simulink model "GFM_GFL_referenceModel_abcCoordinates"  (R2023b)
settings: Solver=ode23  StartTime=0.0  StopTime=SimulationSetup.Solver.timeSimulationEnd  MaxStep=SimulationSetup.Solver.MaxStep  RelTol=SimulationSetup.Solver.RelTol
undefined symbols (not defined in the file): freq, H, Ibase, K_damping, Kdroop_V, Ki_CC, ki_P, ki_PLL, ki_Q, Kp_CC, kp_P, kp_PLL, kp_Q, Lconv1, Lg, Lv, Qref, Rconv1, Rg, Rv, Sbase, SimulationSetup, Vpeak, wf_PQ, wg
libraries: spsPower3phInstantaneousLib x4, eeTransforms x2, eeStairGenerator x1
settings Model: Creator=kauchr  LastModifiedBy=kauchr
settings DataIOCC: SaveFinalState=on  SaveOperatingPoint=on  SaveState=on

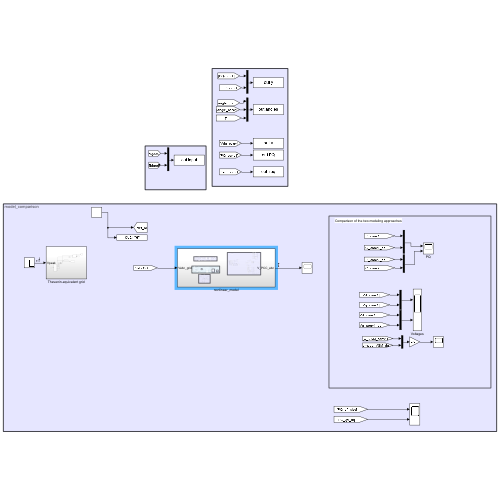
[thumbnail: Simulink's stored preview of the top-level diagram]
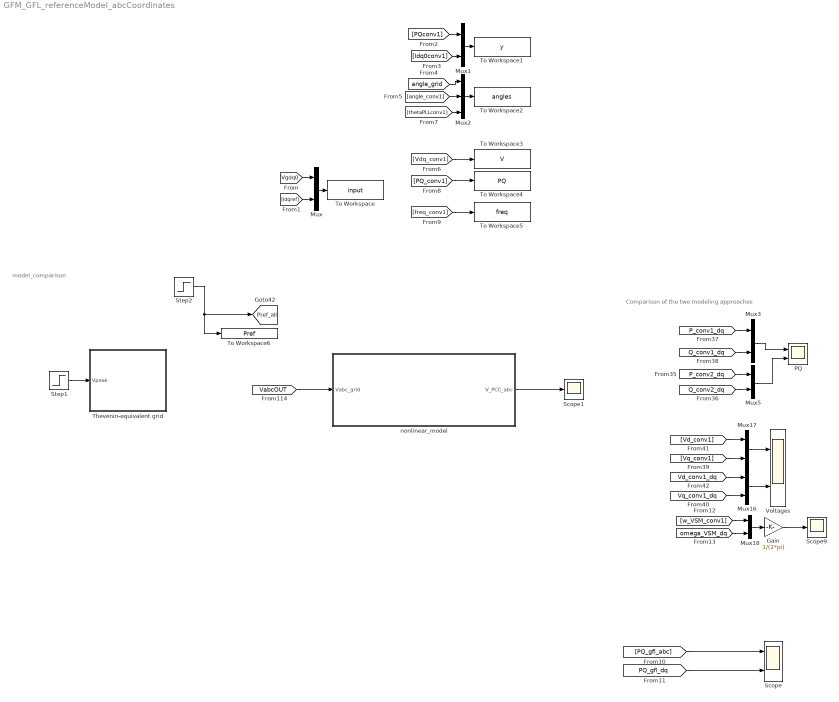
== system GFM_GFL_referenceModel_abcCoordinates ==
  note: model_comparison
  note: Comparison of the two modeling approaches
  Gain : Gain  Gain=1/(2*pi)
  Mux{,1,3,5,16..18} (7 alike) : Mux  Inputs=2
  Mux2 : Mux  Inputs=3
  PQ : Scope  NumInputPorts=2
  Scope : Scope  NumInputPorts=2
  Scope1 : Scope
  Scope9 : Scope
  Step1 : Step  Time=SimulationSetup.grid.voltageAmplitudeStep.Time  Before=SimulationSetup.grid.voltageAmplitudeStep.Values(1)  After=SimulationSetup.grid.voltageAmplitudeStep.Values(2)  SampleTime=0
  Step2 : Step  Time=SimulationSetup.converter1.Pref.Time  Before=SimulationSetup.converter1.Pref.Values(1)  After=SimulationSetup.converter1.Pref.Values(2)  SampleTime=0
  Thevenin-equivalent grid : Subsystem
  To Workspace : ToWorkspace  VariableName=input  SaveFormat=Timeseries  SampleTime=-1
  To Workspace1 : ToWorkspace  VariableName=y  SaveFormat=Timeseries  SampleTime=-1
  To Workspace2 : ToWorkspace  VariableName=angles  SaveFormat=Timeseries  SampleTime=-1
  To Workspace3 : ToWorkspace  VariableName=V  SaveFormat=Timeseries  SampleTime=-1
  To Workspace4 : ToWorkspace  VariableName=PQ  SaveFormat=Timeseries  SampleTime=-1
  To Workspace5 : ToWorkspace  VariableName=freq  SaveFormat=Timeseries  SampleTime=-1
  To Workspace6 : ToWorkspace  VariableName=Pref  SaveFormat=Timeseries  SampleTime=-1
      settings: Save2DSignal=2-D array (concatenate along first dimension)
  Voltages : Scope  NumInputPorts=2
  nonlinear_model : Subsystem
  tag scope: Pref_all=global
  wires:
  [Vgdq0] -> Mux/1
  [Idqref] -> Mux/2
  Mux/1 -> To Workspace/1
  Mux1/1 -> To Workspace1/1
  [PQconv1] -> Mux1/1
  [Idq0conv1] -> Mux1/2
  Mux2/1 -> To Workspace2/1
  [angle_grid] -> Mux2/1
  [angle_conv1] -> Mux2/2
  [Vdq_conv1] -> To Workspace3/1
  [thetaPLLconv1] -> Mux2/3
  [PQ_conv1] -> To Workspace4/1
  [freq_conv1] -> To Workspace5/1
  nonlinear_model/1(V_PCC_abc) -> Scope1/1
  [VabcOUT] -> nonlinear_model/1(Vabc_grid)
  [PQ_gfl_dq] -> Scope/2
  [PQ_gfl_abc] -> Scope/1
  [Vq_conv1] -> Mux17/2
  [Vd_conv1_dq] -> Mux16/1
  [Vq_conv1_dq] -> Mux16/2
  [Vd_conv1] -> Mux17/1
  [P_conv1_dq] -> Mux3/1
  [Q_conv1_dq] -> Mux3/2
  Mux5/1 -> PQ/2
  [Q_conv2_dq] -> Mux5/2
  [P_conv2_dq] -> Mux5/1
  Mux3/1 -> PQ/1
  Gain/1 -> Scope9/1
  Mux18/1 -> Gain/1
  [omega_VSM_dq] -> Mux18/2
  [w_VSM_conv1] -> Mux18/1
  Mux17/1 -> Voltages/1
  Mux16/1 -> Voltages/2
  Step1/1 -> Thevenin-equivalent grid/1(Vpeak)
  Step2/1 -> [Pref_all], To Workspace6/1

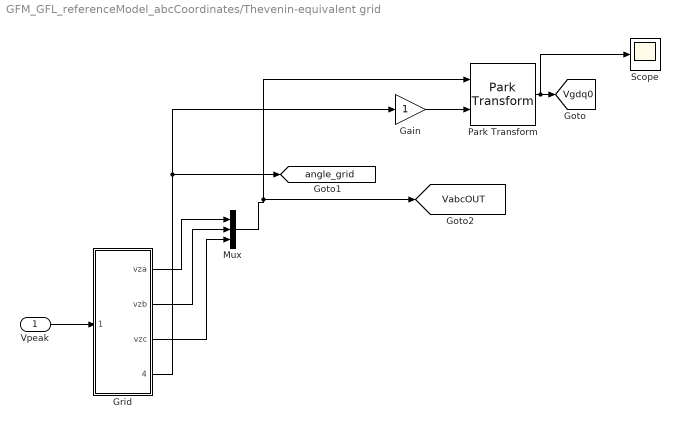
== system GFM_GFL_referenceModel_abcCoordinates/Thevenin-equivalent grid ==
  Vpeak : Inport
  Gain : Gain
  Grid : Subsystem
  Mux : Mux  Inputs=3
  Park Transform : eeTransforms/Park Transform  AxisAlignment=D-axis  PowerInvariant=off
      settings: LibrarySourceBlock=|
      | ee_sl_lib/Mathematical
      | Transforms/Park Transform
  Scope : Scope
  tag scope: VabcOUT=global, Vgdq0=global, angle_grid=global
  wires:
  Grid/4(thetareal) -> [angle_grid], Gain/1
  Grid/2(vzb) -> Mux/2
  Grid/3(vzc) -> Mux/3
  Mux/1 -> Park Transform/1, [VabcOUT]
  Park Transform/1 -> Scope/1, [Vgdq0]
  Grid/1(vza) -> Mux/1
  Vpeak/1 -> Grid/1(Vpeak)
  Gain/1 -> Park Transform/2

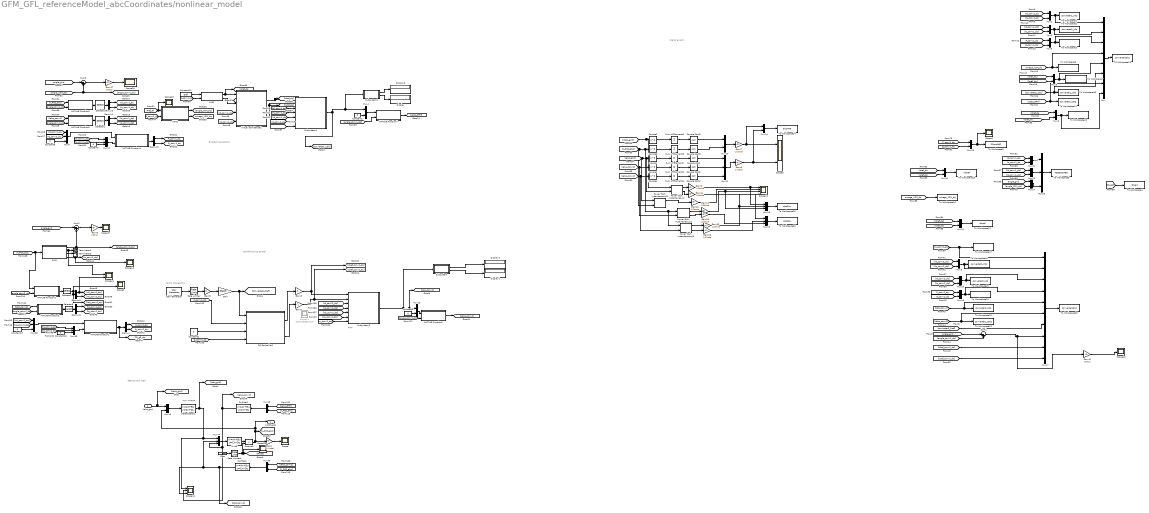
== system GFM_GFL_referenceModel_abcCoordinates/nonlinear_model ==
  note: Grid-forming Control
  note: sign!
  note: had to change this
  note: sign omega
  note: Grid-following Control
  note: Signal export
  note: Network and load
  Vabc_grid : Inport
  AVR2 : Subsystem
  Constant{1..3,6..7,16..17} (7 alike) : Constant  Value=0
  Constant11 : Constant  Value=Qref
  Demux{,1..3,5..6} (6 alike) : Demux  Outputs=2
  Display{,1..3} (4 alike) : Display
  Gain : Gain  Gain=Sbase
  Gain{9..10,12..16} (7 alike) : Gain  Gain=1/Sbase
  Gain11 : Gain  Gain=180/pi
  Gain17 : Gain  Gain=180/pi
  Gain2 : Gain  Gain=-1
  Gain3 : Gain
  Gain4 : Gain  Gain=1/Vpeak
  Gain5 : Gain
  Gain6 : Gain  Gain=180/pi
  Gain7 : Gain  Gain=1/Vpeak
  Gain8 : Gain  Gain=1/Ibase
  MATLAB Function1 : MATLAB Function  TreatAsAtomicUnit=on
  MATLAB Function2 : MATLAB Function  TreatAsAtomicUnit=on
  MATLAB Function3 : MATLAB Function  TreatAsAtomicUnit=on
  MATLAB Function4 : MATLAB Function  TreatAsAtomicUnit=on
  MATLAB Function5 : MATLAB Function  TreatAsAtomicUnit=on
  MATLAB Function6 : MATLAB Function  TreatAsAtomicUnit=on
  MATLAB Function7 : MATLAB Function  TreatAsAtomicUnit=on
  MATLAB Function8 : MATLAB Function  TreatAsAtomicUnit=on
  Mux : Mux  Inputs=[2 2 2 1 2 2 3 2]
  Mux{1..3,5..6,9..10,15..16,21,23..24,29..31} (15 alike) : Mux  Inputs=2
  Mux{8,11..12,18..19,25,38..39} (8 alike) : Mux  Inputs=3
  Mux13 : Mux  Inputs=[2 1]
  Mux14 : Mux  Inputs=[2 3]
  Mux17 : Mux  Inputs=[1 2 2 2 2 3 1 1 1 1]
  Mux4 : Mux  Inputs=[2 1]
  Mux43 : Mux  Inputs=[3 3]
  Mux44 : Mux  Inputs=[3 3 3]
  Mux45 : Mux  Inputs=[3 3]
  Mux46 : Mux  Inputs=[3 3]
  PLL3 : Subsystem
  PQ-Controller2 : Subsystem
  Power (3ph, Instantaneous){,1..3} (4 alike) : spsPower3phInstantaneousLib/Power (3ph, Instantaneous)
  Product1 : Product
  RL-filter1 : StateSpace  A=-Rconv1/Lconv1*eye(3)  B=1/Lconv1*[eye(3),- eye(3)]  C=eye(3)  D=zeros(3,6)  InitialCondition=0
  RL-filter2 : StateSpace  A=-Rconv1/Lconv1*eye(3)  B=1/Lconv1*[eye(3),- eye(3)]  C=eye(3)  D=zeros(3,6)  InitialCondition=0
  Rate Limiter : RateLimiter  RisingSlewLimit=100  FallingSlewLimit=-100  SampleTimeMode=inherited
  Rate Limiter1 : RateLimiter  RisingSlewLimit=1000000  FallingSlewLimit=-1000000  SampleTimeMode=inherited
  Rvirt3 : StateSpace  A=[]  B=[]  C=[]  D=[eye(3),eye(3),eye(3)]  InitialCondition=0  ContinuousStateAttributes='VDQ_PCC'
  Scope{,1,10,13,15..18} (8 alike) : Scope
  Scope11 : Scope  NumInputPorts=3
  Scope12 : Scope  NumInputPorts=4
  Scope14 : Scope  Commented=on  NumInputPorts=2
  Scope2 : Scope  NumInputPorts=2
  Scope24 : Scope  NumInputPorts=2
  Scope3 : Scope  NumInputPorts=2
  Selector{,1..3} (4 alike) : Selector  InputPortWidth=3  IndexOptions=Index vector (dialog)  Indices=[1 2]  OutputSizes=1
  Square{,1..4} (5 alike) : Math  Operator=square
  Square Root{,1..4} (5 alike) : Sqrt
  Stair Generator : eeStairGenerator/Stair Generator  LabelModeActiveChoice=Continuous  TimeInput=SimulationSetup.converter2.Pref.Time  AmplitudeInput=SimulationSetup.converter2.Pref.Values  SampleTime=0  RepeatPattern=off  OutDataTypeStr=double
      settings: LibrarySourceBlock=ee_sl_lib/General Control/Stair Generator
  State-Space1 : StateSpace  A=-Rg/Lg*eye(3)  B=1/Lg*[eye(3),- eye(3)]  C=eye(3)  D=zeros(3,6)  InitialCondition=0
  Step : Step  Time=SimulationSetup.Load.Step.Time  Before=SimulationSetup.Load.Base  After=SimulationSetup.Load.Step.Value  SampleTime=0
  Subsystem : Subsystem
  Subsystem1 : Subsystem
  Subsystem2 : Subsystem
  Subsystem3 : Subsystem
  Sum of Elements{,1..4} (5 alike) : Sum  Inputs=+
  Sum1 : Sum  Inputs=|-+
  Sum2 : Sum  Inputs=|-+
  Sum3 : Sum  Inputs=|-+
  Terminator4 : Terminator
  Terminator5 : Terminator
  To Workspace1 : ToWorkspace  VariableName=converter1_Vdq  SaveFormat=Structure With Time  SampleTime=-1
  To Workspace10 : ToWorkspace  VariableName=Vdqref  SaveFormat=Timeseries  SampleTime=-1
      settings: Save2DSignal=2-D array (concatenate along first dimension)
  To Workspace11 : ToWorkspace  VariableName=Idqref  SaveFormat=Timeseries  SampleTime=-1
      settings: Save2DSignal=2-D array (concatenate along first dimension)
  To Workspace12 : ToWorkspace  VariableName=omega_VSM_dq  SaveFormat=Timeseries  SampleTime=-1
      settings: Save2DSignal=2-D array (concatenate along first dimension)
  To Workspace13 : ToWorkspace  VariableName=converter1_Udq  SaveFormat=Timeseries  SampleTime=-1
      settings: Save2DSignal=2-D array (concatenate along first dimension)
  To Workspace14 : ToWorkspace  VariableName=converter1_UDQ  SaveFormat=Timeseries  SampleTime=-1
      settings: Save2DSignal=2-D array (concatenate along first dimension)
  To Workspace15 : ToWorkspace  VariableName=converter1_Vdrefqref  SaveFormat=Timeseries  SampleTime=-1
      settings: Save2DSignal=2-D array (concatenate along first dimension)
  To Workspace16 : ToWorkspace  VariableName=converter1abc  SaveFormat=Structure With Time  SampleTime=-1
  To Workspace17 : ToWorkspace  VariableName=converter2_omegaPLL  SaveFormat=Timeseries  SampleTime=-1
      settings: Save2DSignal=2-D array (concatenate along first dimension)
  To Workspace18 : ToWorkspace  VariableName=converter2_Vdq  SaveFormat=Structure With Time  SampleTime=-1
  To Workspace19 : ToWorkspace  VariableName=converter2_Idq  SaveFormat=Structure With Time  SampleTime=-1
  To Workspace2 : ToWorkspace  VariableName=converter1_Idq  SaveFormat=Structure With Time  SampleTime=-1
  To Workspace20 : ToWorkspace  VariableName=converter2_PmeasQmeas  SaveFormat=Structure With Time  SampleTime=-1
  To Workspace21 : ToWorkspace  VariableName=converter2_Udq  SaveFormat=Timeseries  SampleTime=-1
      settings: Save2DSignal=2-D array (concatenate along first dimension)
  To Workspace22 : ToWorkspace  VariableName=converter2_Uabc  SaveFormat=Timeseries  SampleTime=-1
      settings: Save2DSignal=2-D array (concatenate along first dimension)
  To Workspace23 : ToWorkspace  VariableName=converter2abc  SaveFormat=Structure  SampleTime=-1
      settings: Save2DSignal=2-D array (concatenate along first dimension)
  To Workspace24 : ToWorkspace  VariableName=abcMAG  SaveFormat=Structure  SampleTime=-1
      settings: Save2DSignal=2-D array (concatenate along first dimension)
  To Workspace25 : ToWorkspace  VariableName=abcPpu  SaveFormat=Structure  SampleTime=-1
      settings: Save2DSignal=2-D array (concatenate along first dimension)
  To Workspace26 : ToWorkspace  VariableName=abcQpu  SaveFormat=Structure  SampleTime=-1
      settings: Save2DSignal=2-D array (concatenate along first dimension)
  To Workspace3 : ToWorkspace  VariableName=converter1_PmeasQmeas  SaveFormat=Structure With Time  SampleTime=-1
  To Workspace4 : ToWorkspace  VariableName=Rload  SaveFormat=Timeseries  SampleTime=-1
      settings: Save2DSignal=2-D array (concatenate along first dimension)
  To Workspace5 : ToWorkspace  VariableName=testDataABC  SaveFormat=Structure With Time  SampleTime=-1
  To Workspace6 : ToWorkspace  VariableName=converter1_omegaVSM  SaveFormat=Timeseries  SampleTime=-1
      settings: Save2DSignal=2-D array (concatenate along first dimension)
  To Workspace7 : ToWorkspace  VariableName=converter1_IdrefIqref  SaveFormat=Timeseries  SampleTime=-1
      settings: Save2DSignal=2-D array (concatenate along first dimension)
  To Workspace9 : ToWorkspace  VariableName=PQoutABC  SaveFormat=Timeseries  SampleTime=-1
      settings: Save2DSignal=2-D array (concatenate along first dimension)
  VSM2 : Subsystem
  Virtual admittance1 : Subsystem
  V_PCC_abc : Outport
  tag scope: PQ_gfl_dq=global, P_conv1_dq=global, P_conv2_dq=global, Q_conv1_dq=global, Q_conv2_dq=global, Vd_conv1_dq=global, Vdref_dq=global, Vq_conv1_dq=global, Vqref_dq=global, omega_VSM_dq=global
  wires:
  [Id_conv1_dq] -> Subsystem1/3(Id)
  Mux24/1 -> Mux25/3
  [Pref_all] -> Scope18/1, VSM2/1(Pref)
  Mux29/1 -> Scope1/1, To Workspace9/1
  Mux30/1 -> To Workspace10/1
  Demux3/2 -> [Q_conv1_dq]
  Constant6/1 -> Mux8/3
  AVR2/1(Vdref) -> [Vdref_dq], Virtual admittance1/1(Vdref)
  [P_conv1_dq] -> VSM2/2(Pmeas)
  [Iq_conv1_dq] -> Mux23/2
  Demux3/1 -> [P_conv1_dq]
  [Vq_conv1_dq] -> Subsystem1/6(Vq)
  [angle_VSM_dq] -> Mux24/2
  Mux31/1 -> To Workspace11/1
  Sum3/1 -> Gain17/1
  [Q_conv1_dq] -> Mux29/2
  [Vd_conv1_dq] -> Mux8/1
  Mux8/1 -> MATLAB Function4/1(Vdq0)
  Constant7/1 -> Mux12/3
  Constant11/1 -> AVR2/1(Qref)
  Virtual admittance1/1(Idref) -> [Idref_dq], Subsystem1/1(Idref)
  [Vq_conv1_dq] -> Mux21/2
  AVR2/2(Vqref) -> [Vqref_dq], Virtual admittance1/2(Vqref)
  Demux1/1 -> [Id_conv1_dq]
  [Id_conv1_dq] -> Mux12/1
  [omega_VSM_dq] -> Subsystem1/7(omega)
  VSM2/1(angle_VSM) -> [angle_VSM_dq]
  [Vq_conv1_dq] -> Mux8/2
  Demux2/2 -> [Vq_conv1_dq]
  Demux1/2 -> [Iq_conv1_dq]
  [Iqref_dq] -> Mux31/2
  [Vd_conv1_dq] -> Subsystem1/5(Vd)
  [Vdref_dq] -> Mux30/1
  [omega_VSM_dq] -> To Workspace12/1
  [Vd_conv1_dq] -> Virtual admittance1/3(Vd)
  [angle_grid] -> Sum3/1
  Demux2/1 -> [Vd_conv1_dq]
  [Q_conv1_dq] -> AVR2/2(Qmeas)
  [Vq_conv1_dq] -> Virtual admittance1/4(Vq)
  Mux23/1 -> Mux25/2
  [Iq_conv1_dq] -> Subsystem1/4(Iq)
  [angle_grid] -> Mux24/1
  [Id_conv1_dq] -> Mux23/1
  Mux21/1 -> Mux25/1
  [Vd_conv1_dq] -> Mux21/1
  [Iq_conv1_dq] -> Mux12/2
  VSM2/2(omega_VSM) -> [omega_VSM_dq]
  [Idref_dq] -> Mux31/1
  Mux25/1 -> To Workspace5/1
  [Vqref_dq] -> Mux30/2
  Virtual admittance1/2(Iqref) -> Subsystem1/2(Iqref), [Iqref_dq]
  [P_conv1_dq] -> Mux29/1
  Subsystem1/1(Uconv_dq) -> [converter1_Udq], Subsystem2/1(dq), Mux4/1
  [Vd_conv2_dq] -> Mux38/1
  MATLAB Function1/1(y) -> [PQ_gfl_dq], Demux/1
  Constant17/1 -> Mux38/3
  Mux38/1 -> MATLAB Function1/1(Vdq0)
  PLL3/2(Vd) -> Scope24/1, Terminator4/1
  Demux6/1 -> [Id_conv2_dq]
  Demux5/2 -> [Vq_conv2_dq]
  [P_conv2_dq] -> PQ-Controller2/2(Pmeas)
  Constant16/1 -> Mux39/3
  Selector2/1 -> [Vdq_conv2_dq], Demux5/1, Scope2/2
  PLL3/1(angle) -> Sum2/2, [angle_conv2_dq]
  [Id_conv2_dq] -> Subsystem3/3(Id)
  [Vq_conv2_dq] -> Mux38/2
  [Id_conv2_dq] -> Mux39/1
  [Iq_conv2_dq] -> Mux39/2
  [Iq_conv2_dq] -> Subsystem3/4(Iq)
  [Q_conv2_dq] -> PQ-Controller2/4(Qmeas)
  PLL3/3(Vq) -> Terminator5/1
  [Vd_conv2_dq] -> Subsystem3/5(Vd)
  [Vq_conv2_dq] -> Subsystem3/6(Vq)
  Demux5/1 -> Scope24/2, [Vd_conv2_dq]
  PLL3/4(w_grid) -> Scope13/1, [w_conv2_dq]
  Demux6/2 -> [Iq_conv2_dq]
  Mux39/1 -> MATLAB Function1/2(Idq0)
  Mux45/1 -> State-Space1/1
  Mux43/1 -> RL-filter2/1
  RL-filter2/1 -> Mux44/3, Scope11/2, [Iabc_conv1]
  [V_PCC_abc] -> Mux46/2
  [Uabc_conv2] -> Mux46/1
  State-Space1/1 -> [Iabc_grid], Scope11/1, Mux44/1
  Mux46/1 -> RL-filter1/1
  Mux44/1 -> Rvirt3/1
  [Uabc_GFM] -> Mux43/1
  [V_PCC_abc] -> Mux43/2
  [w_conv2_dq] -> Subsystem3/7(omega)
  Mux1/1 -> Mux/1, To Workspace1/1
  [Vq_conv1_dq] -> Mux1/2
  [Vd_conv1_dq] -> Mux1/1
  [Iq_conv1_dq] -> Mux2/2
  [Id_conv1_dq] -> Mux2/1
  Mux3/1 -> Mux/3, To Workspace3/1
  [Q_conv1_dq] -> Mux3/2
  [P_conv1_dq] -> Mux3/1
  [omega_VSM_dq] -> Mux/4, To Workspace6/1
  [Idref_dq] -> Mux5/1
  [Iqref_dq] -> Mux5/2
  Mux5/1 -> Mux/5, To Workspace7/1
  [converter1_Udq] -> Mux/6, To Workspace13/1
  [Uabc_GFM] -> Mux/7, To Workspace14/1
  Mux6/1 -> To Workspace15/1, Mux/8
  [Vqref_dq] -> Mux6/2
  [Vdref_dq] -> Mux6/1
  Mux2/1 -> Mux/2, To Workspace2/1
  Mux/1 -> To Workspace16/1
  [w_conv2_dq] -> Mux17/1, To Workspace17/1
  [Vd_conv2_dq] -> Mux9/1
  Mux9/1 -> Mux17/2, To Workspace18/1
  Mux15/1 -> Mux17/3, To Workspace19/1
  [P_conv2_dq] -> Mux16/1
  [Vq_conv2_dq] -> Mux9/2
  Mux16/1 -> Mux17/4, To Workspace20/1
  [Q_conv2_dq] -> Mux16/2
  [Iq_conv2_dq] -> Mux15/2
  [Id_conv2_dq] -> Mux15/1
  [Udq_conv2] -> Mux17/5, To Workspace21/1
  [Uabc_conv2] -> Mux17/6, To Workspace22/1
  Mux17/1 -> To Workspace23/1
  Vabc_grid/1 -> [Vabc_grid], Mux45/1
  Selector3/1 -> Demux6/1
  [V_PCC_abc] -> MATLAB Function5/1(Vabc)
  [angle_conv1_dq] -> MATLAB Function5/2(theta)
  Selector1/1 -> Demux1/1
  [Iabc_conv1] -> MATLAB Function6/1(Vabc)
  [angle_conv1_dq] -> MATLAB Function6/2(theta)
  Selector/1 -> Demux2/1
  Stair Generator/1 -> Rate Limiter/1
  PQ-Controller2/1(Idref) -> Gain3/1
  PQ-Controller2/2(Iqref) -> Gain2/1
  Gain3/1 -> [Idref_conv2_dq], Subsystem3/1(Idref)
  Gain2/1 -> Subsystem3/2(Iqref), [Iqref_conv2_dq]
  Constant2/1 -> PQ-Controller2/3(Qref)
  [converter2_Pref] -> Mux17/7
  Rate Limiter/1 -> Gain5/1
  RL-filter1/1 -> Mux44/2, Scope11/3, [Iabc_conv2]
  [Idref_conv2_dq] -> Mux17/9
  [Iqref_conv2_dq] -> Mux17/10
  Rvirt3/1 -> Product1/1
  Product1/1 -> Gain4/1, Mux45/2, V_PCC_abc/1, [V_PCC_abc]
  Step/1 -> Rate Limiter1/1
  Gain4/1 -> Scope/1
  [Rload] -> To Workspace4/1
  Rate Limiter1/1 -> Product1/2, [Rload], Scope15/1
  Gain5/1 -> Gain/1
  Gain6/1 -> Scope17/1
  Gain7/1 -> Mux14/1, Scope3/1
  Square Root3/1 -> Mux10/2  "load"
  Square Root1/1 -> Mux11/2  "GFL"
  Square Root2/1 -> Mux10/1  "grid"
  Gain8/1 -> Mux14/2, Scope3/2
  [V_PCC_abc] -> "Power (3ph, Instantaneous)3"/1, "Power (3ph, Instantaneous)2"/1, Square3/1, "Power (3ph, Instantaneous)1"/2
  [Iabc_grid] -> "Power (3ph, Instantaneous)"/2, Square/1, "Power (3ph, Instantaneous)1"/1
  Sum of Elements3/1 -> Square Root3/1
  Square3/1 -> Sum of Elements3/1
  Square2/1 -> Sum of Elements2/1
  [Iabc_conv2] -> "Power (3ph, Instantaneous)2"/2, Square1/1
  Sum of Elements2/1 -> Square Root2/1
  Square Root/1 -> Mux11/1  "grid"
  Square1/1 -> Sum of Elements1/1
  Square/1 -> Sum of Elements/1
  Sum of Elements/1 -> Square Root/1
  Mux11/1 -> Gain8/1
  [Vabc_grid] -> "Power (3ph, Instantaneous)"/1, Square2/1
  Mux10/1 -> Gain7/1
  Sum of Elements1/1 -> Square Root1/1
  Square4/1 -> Sum of Elements4/1
  Sum of Elements4/1 -> Square Root4/1
  [Iabc_conv1] -> "Power (3ph, Instantaneous)3"/2, Square4/1
  Square Root4/1 -> Mux11/3  "GFM"
  MATLAB Function5/1(y) -> Selector/1
  MATLAB Function6/1(y) -> Selector1/1
  [angle_conv1_dq] -> MATLAB Function7/2(theta)
  Mux4/1 -> MATLAB Function7/1(Vdq0)
  Constant1/1 -> Mux4/2
  [angle_VSM_dq] -> [angle_conv1_dq], Sum3/2
  [angle_conv2_dq] -> MATLAB Function3/2(theta)
  [Iabc_conv2] -> MATLAB Function3/1(Iabc)
  MATLAB Function2/1(y) -> Selector2/1
  [angle_conv2_dq] -> MATLAB Function2/2(theta)
  MATLAB Function3/1(y) -> Selector3/1
  [V_PCC_abc] -> MATLAB Function2/1(Vabc), PLL3/1(Vabc)
  Constant3/1 -> Mux13/2
  [angle_conv2_dq] -> MATLAB Function8/2(theta)
  MATLAB Function8/1(Vabc) -> [Uabc_conv2]
  Mux13/1 -> MATLAB Function8/1(Vdq0)
  Mux14/1 -> To Workspace24/1
  [angle_grid] -> Sum1/1
  [angle_conv2_dq] -> Sum1/2
  Sum1/1 -> Gain11/1, Mux17/8
  "Power (3ph, Instantaneous)"/1 -> Gain9/1
  "Power (3ph, Instantaneous)1"/1 -> Gain10/1
  Gain9/1 -> Mux18/1, Scope12/1
  Gain10/1 -> Scope12/2
  Gain11/1 -> Scope10/1
  "Power (3ph, Instantaneous)2"/1 -> Gain12/1
  Gain12/1 -> Mux18/3, Scope12/3
  "Power (3ph, Instantaneous)3"/1 -> Gain13/1
  Gain13/1 -> Mux18/2, Scope12/4
  Mux18/1 -> To Workspace25/1
  "Power (3ph, Instantaneous)"/2 -> Gain14/1
  Mux19/1 -> To Workspace26/1
  Gain14/1 -> Mux19/1
  "Power (3ph, Instantaneous)2"/2 -> Gain15/1
  "Power (3ph, Instantaneous)3"/2 -> Gain16/1
  Gain16/1 -> Mux19/2
  Gain15/1 -> Mux19/3
  Subsystem3/1(Uconv_dq) -> Subsystem/1(dq), Mux13/1, [Udq_conv2]
  Subsystem/1(Vmag (pu)) -> Display2/1
  Subsystem/2(Angle (°)) -> Display1/1
  Subsystem2/2(Angle (°)) -> Display/1
  Subsystem2/1(Vmag (pu)) -> Display3/1
  Gain17/1 -> Scope16/1
  [angle_grid] -> Sum2/1
  Sum2/1 -> Gain6/1
  Gain/1 -> [converter2_Pref], PQ-Controller2/1(Pref)
  Demux/1 -> [P_conv2_dq]
  Demux/2 -> [Q_conv2_dq]
  Mux12/1 -> MATLAB Function4/2(Idq0)
  MATLAB Function4/1(y) -> Demux3/1
  MATLAB Function7/1(Vabc) -> [Uabc_GFM]

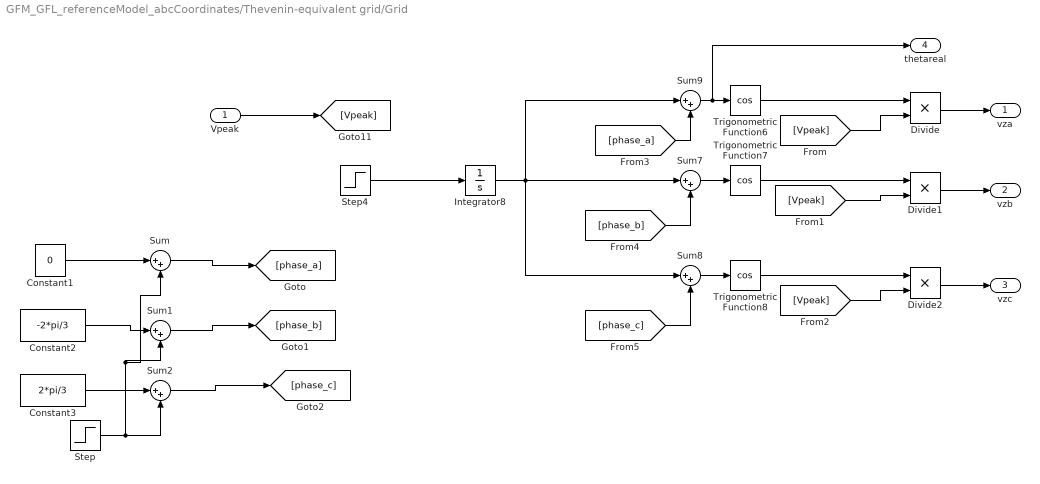
== system GFM_GFL_referenceModel_abcCoordinates/Thevenin-equivalent grid/Grid ==
  Vpeak : Inport
  Constant1 : Constant  Value=0
  Constant2 : Constant  Value=-2*pi/3
  Constant3 : Constant  Value=2*pi/3
  Divide : Product  Inputs=**
  Divide1 : Product  Inputs=**
  Divide2 : Product  Inputs=**
  Integrator8 : Integrator  ContinuousStateAttributes='grid_thetaGRID'
  Step : Step  Time=SimulationSetup.grid.PhaseStep.Time  Before=SimulationSetup.grid.PhaseStep.Values(1)  After=SimulationSetup.grid.PhaseStep.Values(2)  SampleTime=0
  Step4 : Step  Time=SimulationSetup.grid.FrequencyStep.Time  Before=SimulationSetup.grid.FrequencyStep.Values(1)  After=SimulationSetup.grid.FrequencyStep.Values(2)  SampleTime=0
  Sum{,1..2,7..9} (6 alike) : Sum  Inputs=|++
  Trigonometric Function6 : Trigonometry  Operator=cos
  Trigonometric Function7 : Trigonometry  Operator=cos
  Trigonometric Function8 : Trigonometry  Operator=cos
  vza : Outport
  vzb : Outport  Port=2
  vzc : Outport  Port=3
  thetareal : Outport  Port=4
  wires:
  Sum9/1 -> thetareal/1, Trigonometric Function6/1
  [phase_c] -> Sum8/2
  Integrator8/1 -> Sum8/1, Sum9/1, Sum7/1
  [phase_b] -> Sum7/2
  Sum7/1 -> Trigonometric Function7/1
  [phase_a] -> Sum9/2
  Sum8/1 -> Trigonometric Function8/1
  Trigonometric Function6/1 -> Divide/1
  Trigonometric Function7/1 -> Divide1/1
  Trigonometric Function8/1 -> Divide2/1
  Divide/1 -> vza/1
  Divide1/1 -> vzb/1
  Divide2/1 -> vzc/1
  [Vpeak] -> Divide/2
  [Vpeak] -> Divide1/2
  [Vpeak] -> Divide2/2
  Sum1/1 -> [phase_b]
  Sum/1 -> [phase_a]
  Constant1/1 -> Sum/1
  Constant2/1 -> Sum1/1
  Constant3/1 -> Sum2/1
  Sum2/1 -> [phase_c]
  Step/1 -> Sum/2, Sum1/2, Sum2/2
  Step4/1 -> Integrator8/1
  Vpeak/1 -> [Vpeak]

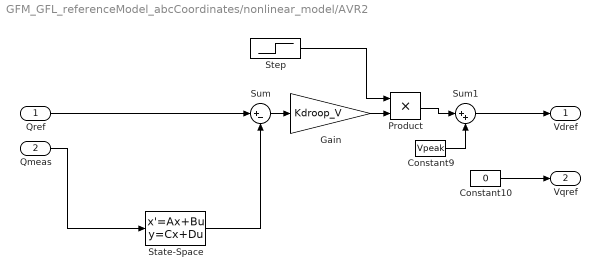
== system GFM_GFL_referenceModel_abcCoordinates/nonlinear_model/AVR2 ==
  Qref : Inport
  Qmeas : Inport  Port=2
  Constant10 : Constant  Value=0
  Constant9 : Constant  Value=Vpeak
  Gain : Gain  Gain=Kdroop_V
  Product : Product
  State-Space : StateSpace  A=-wf_PQ  B=wf_PQ  D=0  InitialCondition=0  ContinuousStateAttributes='converter1_xI_Vdroop'
  Step : Step  Time=SimulationSetup.converter1.VoltageCtrl.ActivationTime  SampleTime=0
  Sum : Sum  Inputs=|+-
  Sum1 : Sum  Inputs=|++
  Vdref : Outport
  Vqref : Outport  Port=2
  wires:
  Qref/1 -> Sum/1
  Constant9/1 -> Sum1/2
  Sum/1 -> Gain/1
  Qmeas/1 -> State-Space/1
  Product/1 -> Sum1/1
  Step/1 -> Product/1
  Gain/1 -> Product/2
  State-Space/1 -> Sum/2
  Sum1/1 -> Vdref/1
  Constant10/1 -> Vqref/1

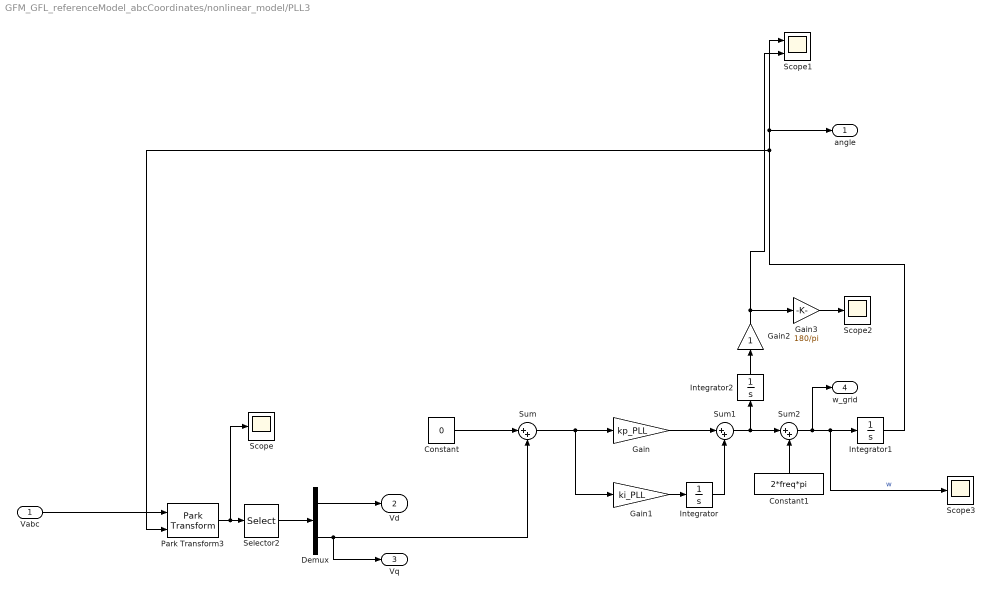
== system GFM_GFL_referenceModel_abcCoordinates/nonlinear_model/PLL3 ==
  Vabc : Inport
  Constant : Constant  Value=0
  Constant1 : Constant  Value=2*freq*pi
  Demux : Demux  Outputs=2
  Gain : Gain  Gain=kp_PLL
  Gain1 : Gain  Gain=ki_PLL
  Gain2 : Gain
  Gain3 : Gain  Gain=180/pi
  Integrator : Integrator  ContinuousStateAttributes='converter2_xI_PLL'
  Integrator1 : Integrator  ContinuousStateAttributes='converter2_thetaPLL'
  Integrator2 : Integrator  ContinuousStateAttributes='converter2_deltaPLL'
  Park Transform3 : eeTransforms/Park Transform  AxisAlignment=D-axis  PowerInvariant=off
      settings: LibrarySourceBlock=|
      | ee_sl_lib/Mathematical
      | Transforms/Park Transform
  Scope : Scope
  Scope1 : Scope  NumInputPorts=2
  Scope2 : Scope
  Scope3 : Scope
  Selector2 : Selector  InputPortWidth=3  IndexOptions=Index vector (dialog)  Indices=[1 2]  OutputSizes=1
  Sum : Sum  Inputs=|++
  Sum1 : Sum  Inputs=|++
  Sum2 : Sum  Inputs=|++
  angle : Outport
  Vd : Outport  Port=2
  Vq : Outport  Port=3
  w_grid : Outport  Port=4
  wires:
  Sum1/1 -> Sum2/1, Integrator2/1
  Gain/1 -> Sum1/1
  Integrator/1 -> Sum1/2
  Gain1/1 -> Integrator/1
  Demux/1 -> Vd/1
  Sum2/1 -> w_grid/1, Scope3/1, Integrator1/1  "w"
  Constant/1 -> Sum/1
  Constant1/1 -> Sum2/2
  Vabc/1 -> Park Transform3/1
  Sum/1 -> Gain1/1, Gain/1
  Demux/2 -> Sum/2, Vq/1
  Integrator2/1 -> Gain2/1
  Integrator1/1 -> Park Transform3/2, angle/1, Scope1/1
  Gain2/1 -> Gain3/1, Scope1/2
  Park Transform3/1 -> Scope/1, Selector2/1
  Selector2/1 -> Demux/1
  Gain3/1 -> Scope2/1

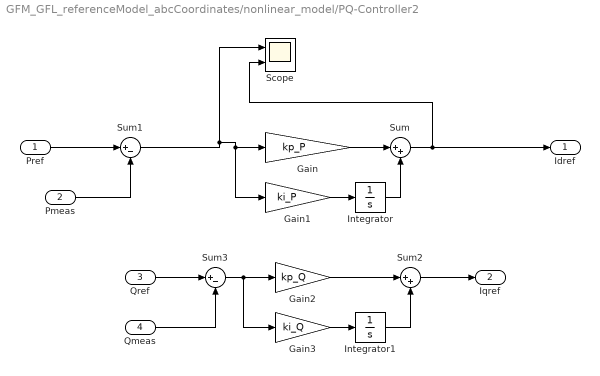
== system GFM_GFL_referenceModel_abcCoordinates/nonlinear_model/PQ-Controller2 ==
  Pref : Inport
  Pmeas : Inport  Port=2
  Qref : Inport  Port=3
  Qmeas : Inport  Port=4
  Gain : Gain  Gain=kp_P
  Gain1 : Gain  Gain=ki_P
  Gain2 : Gain  Gain=kp_Q
  Gain3 : Gain  Gain=ki_Q
  Integrator : Integrator  ContinuousStateAttributes='converter2_xI_Pctrl'
  Integrator1 : Integrator  ContinuousStateAttributes='converter2_xI_Qctrl'
  Scope : Scope  NumInputPorts=2
  Sum : Sum  Inputs=|++
  Sum1 : Sum  Inputs=|+-
  Sum2 : Sum  Inputs=|++
  Sum3 : Sum  Inputs=|+-
  Idref : Outport
  Iqref : Outport  Port=2
  wires:
  Gain1/1 -> Integrator/1
  Integrator/1 -> Sum/2
  Gain/1 -> Sum/1
  Sum/1 -> Idref/1, Scope/2
  Pmeas/1 -> Sum1/2
  Integrator1/1 -> Sum2/2
  Sum2/1 -> Iqref/1
  Sum3/1 -> Gain3/1, Gain2/1
  Gain2/1 -> Sum2/1
  Qmeas/1 -> Sum3/2
  Gain3/1 -> Integrator1/1
  Qref/1 -> Sum3/1
  Sum1/1 -> Scope/1, Gain1/1, Gain/1
  Pref/1 -> Sum1/1

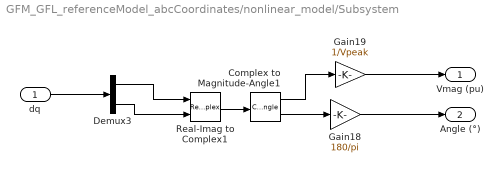
== system GFM_GFL_referenceModel_abcCoordinates/nonlinear_model/Subsystem ==
  dq : Inport
  Complex to Magnitude-Angle1 : ComplexToMagnitudeAngle
  Demux3 : Demux  Outputs=2
  Gain18 : Gain  Gain=180/pi
  Gain19 : Gain  Gain=1/Vpeak
  Real-Imag to Complex1 : RealImagToComplex
  Vmag (pu) : Outport
  Angle (°) : Outport  Port=2
  wires:
  Demux3/2 -> Real-Imag to Complex1/2
  Complex to Magnitude-Angle1/1 -> Gain19/1
  dq/1 -> Demux3/1
  Gain19/1 -> Vmag (pu)/1
  Complex to Magnitude-Angle1/2 -> Gain18/1
  Real-Imag to Complex1/1 -> Complex to Magnitude-Angle1/1
  Gain18/1 -> Angle (°)/1
  Demux3/1 -> Real-Imag to Complex1/1

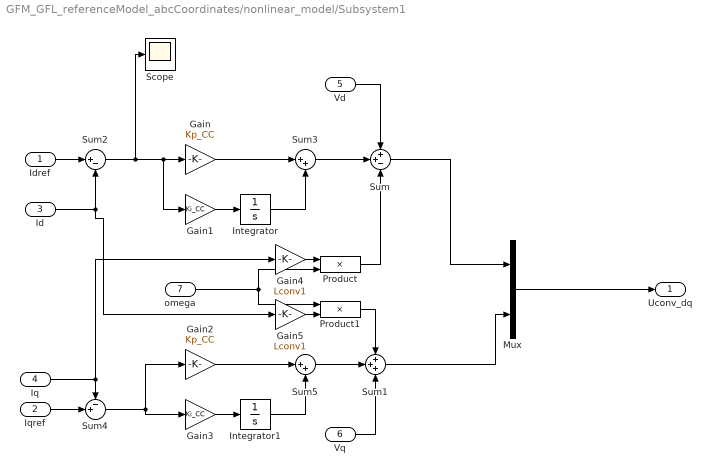
== system GFM_GFL_referenceModel_abcCoordinates/nonlinear_model/Subsystem1 ==
  Idref : Inport
  Iqref : Inport  Port=2
  Id : Inport  Port=3
  Iq : Inport  Port=4
  Vd : Inport  Port=5
  Vq : Inport  Port=6
  omega : Inport  Port=7
  Gain : Gain  Gain=Kp_CC
  Gain1 : Gain  Gain=Ki_CC
  Gain2 : Gain  Gain=Kp_CC
  Gain3 : Gain  Gain=Ki_CC
  Gain4 : Gain  Gain=Lconv1
  Gain5 : Gain  Gain=Lconv1
  Integrator : Integrator  ContinuousStateAttributes='converter1_xId_CC'
  Integrator1 : Integrator  ContinuousStateAttributes='converter1_xIq_CC'
  Mux : Mux  Inputs=2
  Product : Product
  Product1 : Product
  Scope : Scope
  Sum : Sum  Inputs=++-
  Sum1 : Sum  Inputs=+++
  Sum2 : Sum  Inputs=|+-
  Sum3 : Sum  Inputs=|++
  Sum4 : Sum  Inputs=-+|
  Sum5 : Sum  Inputs=|++
  Uconv_dq : Outport
  wires:
  Vd/1 -> Sum/1
  Vq/1 -> Sum1/3
  Sum/1 -> Mux/1
  Sum1/1 -> Mux/2
  Mux/1 -> Uconv_dq/1
  Idref/1 -> Sum2/1
  Id/1 -> Sum2/2, Gain5/1
  Sum2/1 -> Scope/1, Gain1/1, Gain/1
  Gain1/1 -> Integrator/1
  Integrator/1 -> Sum3/2
  Gain/1 -> Sum3/1
  Sum3/1 -> Sum/2
  Iqref/1 -> Sum4/2
  Iq/1 -> Gain4/1, Sum4/1
  Integrator1/1 -> Sum5/2
  Sum5/1 -> Sum1/2
  Gain3/1 -> Integrator1/1
  Gain2/1 -> Sum5/1
  Sum4/1 -> Gain2/1, Gain3/1
  Gain4/1 -> Product/1
  Product/1 -> Sum/3
  omega/1 -> Product/2, Product1/1
  Gain5/1 -> Product1/2
  Product1/1 -> Sum1/1

== system GFM_GFL_referenceModel_abcCoordinates/nonlinear_model/Subsystem2 ==
  dq : Inport
  Complex to Magnitude-Angle1 : ComplexToMagnitudeAngle
  Demux3 : Demux  Outputs=2
  Gain18 : Gain  Gain=180/pi
  Gain19 : Gain  Gain=1/Vpeak
  Real-Imag to Complex1 : RealImagToComplex
  Vmag (pu) : Outport
  Angle (°) : Outport  Port=2
  wires:
  Demux3/2 -> Real-Imag to Complex1/2
  Complex to Magnitude-Angle1/1 -> Gain19/1
  dq/1 -> Demux3/1
  Gain19/1 -> Vmag (pu)/1
  Complex to Magnitude-Angle1/2 -> Gain18/1
  Real-Imag to Complex1/1 -> Complex to Magnitude-Angle1/1
  Gain18/1 -> Angle (°)/1
  Demux3/1 -> Real-Imag to Complex1/1

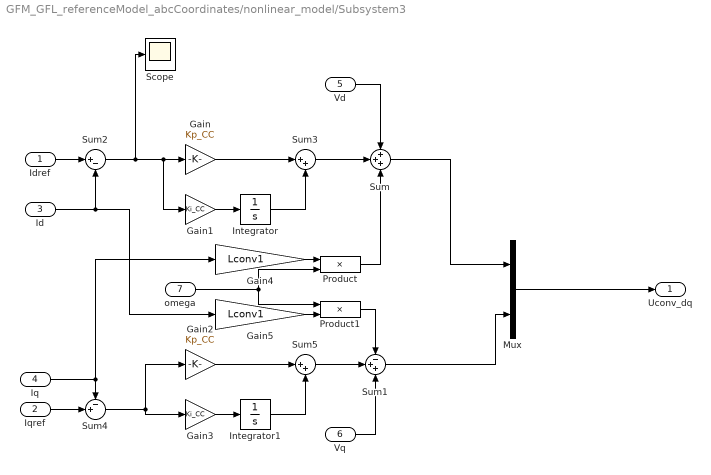
== system GFM_GFL_referenceModel_abcCoordinates/nonlinear_model/Subsystem3 ==
  Idref : Inport
  Iqref : Inport  Port=2
  Id : Inport  Port=3
  Iq : Inport  Port=4
  Vd : Inport  Port=5
  Vq : Inport  Port=6
  omega : Inport  Port=7
  Gain : Gain  Gain=Kp_CC
  Gain1 : Gain  Gain=Ki_CC
  Gain2 : Gain  Gain=Kp_CC
  Gain3 : Gain  Gain=Ki_CC
  Gain4 : Gain  Gain=Lconv1
  Gain5 : Gain  Gain=Lconv1
  Integrator : Integrator  ContinuousStateAttributes='converter2_xId_CC'
  Integrator1 : Integrator  ContinuousStateAttributes='converter2_xIq_CC'
  Mux : Mux  Inputs=2
  Product : Product
  Product1 : Product
  Scope : Scope
  Sum : Sum  Inputs=+++
  Sum1 : Sum  Inputs=-++
  Sum2 : Sum  Inputs=|+-
  Sum3 : Sum  Inputs=|++
  Sum4 : Sum  Inputs=-+|
  Sum5 : Sum  Inputs=|++
  Uconv_dq : Outport
  wires:
  Vd/1 -> Sum/1
  Vq/1 -> Sum1/3
  Sum/1 -> Mux/1
  Sum1/1 -> Mux/2
  Mux/1 -> Uconv_dq/1
  Idref/1 -> Sum2/1
  Id/1 -> Sum2/2, Gain5/1
  Sum2/1 -> Scope/1, Gain1/1, Gain/1
  Gain1/1 -> Integrator/1
  Integrator/1 -> Sum3/2
  Gain/1 -> Sum3/1
  Sum3/1 -> Sum/2
  Iqref/1 -> Sum4/2
  Iq/1 -> Gain4/1, Sum4/1
  Integrator1/1 -> Sum5/2
  Sum5/1 -> Sum1/2
  Gain3/1 -> Integrator1/1
  Gain2/1 -> Sum5/1
  Sum4/1 -> Gain2/1, Gain3/1
  Gain4/1 -> Product/1
  Product/1 -> Sum/3
  omega/1 -> Product/2, Product1/1
  Gain5/1 -> Product1/2
  Product1/1 -> Sum1/1

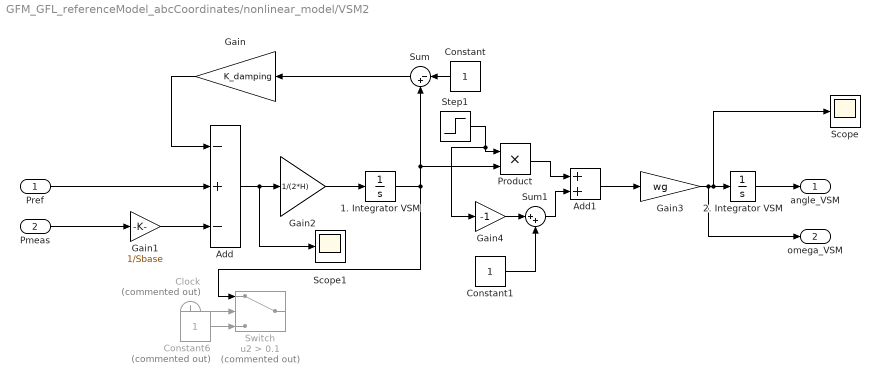
== system GFM_GFL_referenceModel_abcCoordinates/nonlinear_model/VSM2 ==
  Pref : Inport
  Pmeas : Inport  Port=2
  1. Integrator VSM : Integrator  ContinuousStateAttributes='converter1_xI_vsm'
  2. Integrator VSM : Integrator  ContinuousStateAttributes='converter1_thetaVSM'
  Add : Sum  Inputs=-+-
  Add1 : Sum
  Clock : Clock  Commented=on
  Constant : Constant
  Constant1 : Constant
  Constant6 : Constant  Commented=on
  Gain : Gain  Gain=K_damping
  Gain1 : Gain  Gain=1/Sbase
  Gain2 : Gain  Gain=1/(2*H)
  Gain3 : Gain  Gain=wg
  Gain4 : Gain  Gain=-1
  Product : Product
  Scope : Scope
  Scope1 : Scope
  Step1 : Step  Time=SimulationSetup.converter1.FreqCtrl.ActivationTime  SampleTime=0
  Sum : Sum  Inputs=|-+
  Sum1 : Sum  Inputs=|++
  Switch : Switch  Commented=on  Criteria=u2 > Threshold  Threshold=0.1  SaturateOnIntegerOverflow=off  InputSameDT=off
  angle_VSM : Outport
  omega_VSM : Outport  Port=2
  wires:
  Pmeas/1 -> Gain1/1
  Gain2/1 -> 1. Integrator VSM/1
  Pref/1 -> Add/2
  Gain1/1 -> Add/3
  Add/1 -> Scope1/1, Gain2/1
  1. Integrator VSM/1 -> Product/2, Sum/2, Switch/1
  Constant/1 -> Sum/1
  Sum/1 -> Gain/1
  Gain/1 -> Add/1
  Gain3/1 -> omega_VSM/1, Scope/1, 2. Integrator VSM/1
  2. Integrator VSM/1 -> angle_VSM/1
  Clock/1 -> Switch/2
  Constant6/1 -> Switch/3
  Add1/1 -> Gain3/1
  Product/1 -> Add1/1
  Step1/1 -> Gain4/1, Product/1
  Gain4/1 -> Sum1/1
  Sum1/1 -> Add1/2
  Constant1/1 -> Sum1/2

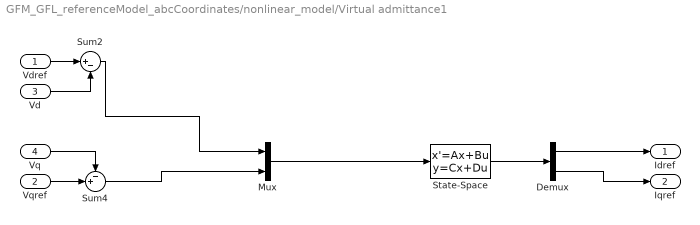
== system GFM_GFL_referenceModel_abcCoordinates/nonlinear_model/Virtual admittance1 ==
  Vdref : Inport
  Vqref : Inport  Port=2
  Vd : Inport  Port=3
  Vq : Inport  Port=4
  Demux : Demux  Outputs=2
  Mux : Mux  Inputs=2
  State-Space : StateSpace  A=[-Rv/Lv, +wg; -wg, -Rv/Lv]  B=[1 0; 0 1]  C=1/Lv*eye(2)  D=zeros(2,2)  InitialCondition=0  ContinuousStateAttributes={'converter1_xId_VA','converter1_xIq_VA'}
  Sum2 : Sum  Inputs=|+-
  Sum4 : Sum  Inputs=-+|
  Idref : Outport
  Iqref : Outport  Port=2
  wires:
  Vdref/1 -> Sum2/1
  Vd/1 -> Sum2/2
  Vqref/1 -> Sum4/2
  Vq/1 -> Sum4/1
  Sum2/1 -> Mux/1
  Sum4/1 -> Mux/2
  Mux/1 -> State-Space/1
  State-Space/1 -> Demux/1
  Demux/1 -> Idref/1
  Demux/2 -> Iqref/1

== matlab function GFM_GFL_referenceModel_abcCoordinates/nonlinear_model/MATLAB Function1 ==
  data: y output; Vdq0 input; Idq0 input
function y= PQcalculation(Vdq0,Idq0)
 % alignment with d-axis
y =3/2*([Vdq0(1)*Idq0(1)+Vdq0(2)*Idq0(2)+2*Vdq0(3)*Idq0(3);Vdq0(2)*Idq0(1)-Vdq0(1)*Idq0(2);]);

== matlab function GFM_GFL_referenceModel_abcCoordinates/nonlinear_model/MATLAB Function3 ==
  data: Iabc input; y output; theta input
function y = abc2dq0(Iabc,theta)
 % alignment with d-axis
y =2/3*([cos(theta), cos(theta-2*pi/3),cos(theta+2*pi/3); -sin(theta), -sin(theta-2*pi/3), -sin(theta+2*pi/3); sqrt(0.5),sqrt(0.5),sqrt(0.5) ])*[Iabc(1);Iabc(2);Iabc(3)];

== matlab function GFM_GFL_referenceModel_abcCoordinates/nonlinear_model/MATLAB Function4 ==
  data: y output; Vdq0 input; Idq0 input
function y= PQcalculation(Vdq0,Idq0)
 % alignment with d-axis
y =3/2*([Vdq0(1)*Idq0(1)+Vdq0(2)*Idq0(2)+2*Vdq0(3)*Idq0(3);Vdq0(2)*Idq0(1)-Vdq0(1)*Idq0(2);]);

== matlab function GFM_GFL_referenceModel_abcCoordinates/nonlinear_model/MATLAB Function5 ==
  data: Vabc input; y output; theta input
function y = abc2dq0(Vabc,theta)
 % alignment with d-axis
y =2/3*([cos(theta), cos(theta-2*pi/3),cos(theta+2*pi/3); -sin(theta), -sin(theta-2*pi/3), -sin(theta+2*pi/3); sqrt(0.5),sqrt(0.5),sqrt(0.5) ])*[Vabc(1);Vabc(2);Vabc(3)];

== matlab function GFM_GFL_referenceModel_abcCoordinates/nonlinear_model/MATLAB Function6 ==
  data: Vabc input; y output; theta input
function y = abc2dq0(Vabc,theta)
 % alignment with d-axis
y =2/3*([cos(theta), cos(theta-2*pi/3),cos(theta+2*pi/3); -sin(theta), -sin(theta-2*pi/3), -sin(theta+2*pi/3); sqrt(0.5),sqrt(0.5),sqrt(0.5) ])*[Vabc(1);Vabc(2);Vabc(3)];

== matlab function GFM_GFL_referenceModel_abcCoordinates/nonlinear_model/MATLAB Function7 ==
  data: Vdq0 input; Vabc output; theta input
function Vabc = dq02abc(Vdq0,theta)
 % alignment with d-axis
Vabc= [cos(theta), -sin(theta), 1; cos(theta-2*pi/3), -sin(theta-2*pi/3), 1;cos(theta+2*pi/3) , -sin(theta+2*pi/3),1;]*[Vdq0(1);Vdq0(2);Vdq0(3)];

== matlab function GFM_GFL_referenceModel_abcCoordinates/nonlinear_model/MATLAB Function8 ==
  data: Vdq0 input; Vabc output; theta input
function Vabc = dq02abc(Vdq0,theta)
 % alignment with d-axis
Vabc= [cos(theta), -sin(theta), 1; cos(theta-2*pi/3), -sin(theta-2*pi/3), 1;cos(theta+2*pi/3) , -sin(theta+2*pi/3),1;]*[Vdq0(1);Vdq0(2);Vdq0(3)];

== matlab function GFM_GFL_referenceModel_abcCoordinates/nonlinear_model/MATLAB Function2 ==
  data: Vabc input; y output; theta input
function y = abc2dq0(Vabc,theta)
 % alignment with d-axis
y =2/3*([cos(theta), cos(theta-2*pi/3),cos(theta+2*pi/3); -sin(theta), -sin(theta-2*pi/3), -sin(theta+2*pi/3); sqrt(0.5),sqrt(0.5),sqrt(0.5) ])*[Vabc(1);Vabc(2);Vabc(3)];
